simulink model "BolandLab3"  (R2024a)
settings: Solver=VariableStepAuto  StartTime=0.0  StopTime=100  RelTol=1e-3
libraries: simulink x1, dspsigops x1
settings Model: Creator=Test  LastModifiedBy=Test

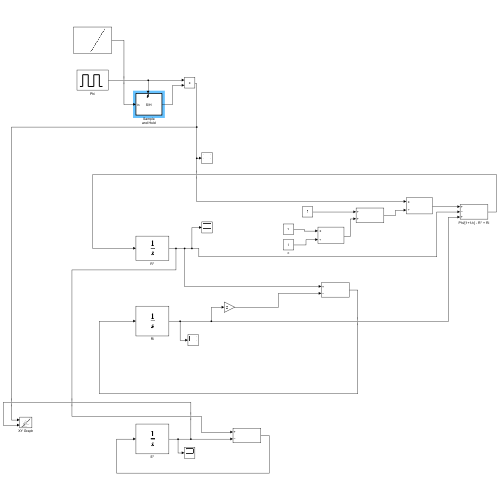
[thumbnail: Simulink's stored preview of the top-level diagram]
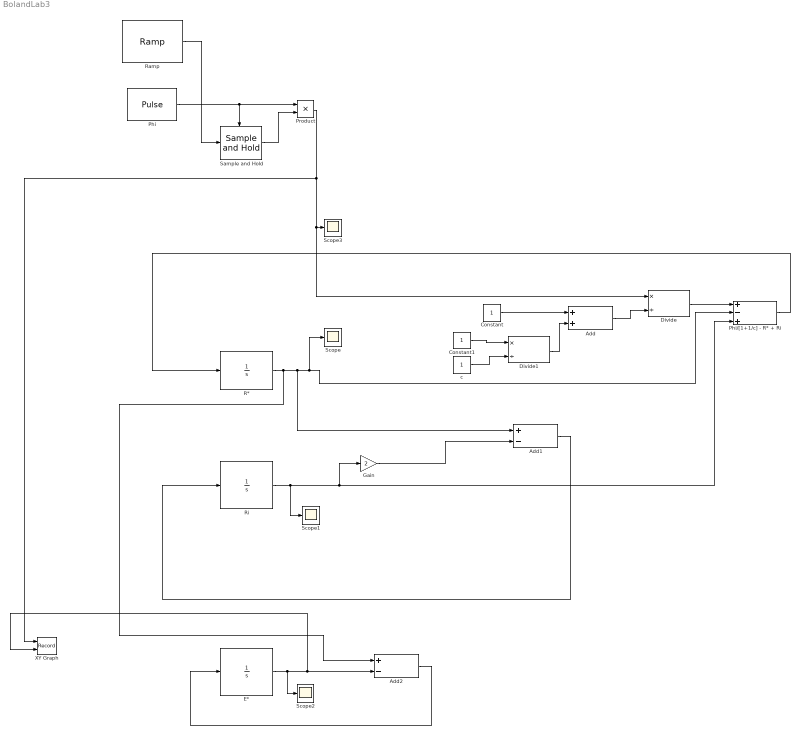
== system BolandLab3 ==
  Add : Sum
  Add1 : Sum  Inputs=+-
  Add2 : Sum  Inputs=+-
  Constant : Constant
  Constant1 : Constant
  Divide : Product  Inputs=*/
  Divide1 : Product  Inputs=*/
  E* : Integrator
  Gain : Gain  Gain=2
  Phi : DiscretePulseGenerator  PulseType=Time based  Period=10
  Phi/[1+1/c] - R* + Ri : Sum  Inputs=+-+
  Product : Product
  R* : Integrator
  Ramp : simulink/Sources/Ramp  slope=.1  start=0  InitialOutput=0
  Ri : Integrator
  Sample and Hold : dspsigops/Sample and Hold  trig=Rising edge  initCond=0  latchinput=off
  Scope{,1..3} (4 alike) : Scope
  XY Graph : Record  FileSettingsInternal="{\"entries\":[{\"content\":{\"excelSettings\":{\"content\":{},\"type\":\"Streamout.ExcelSettings\"}},\"type\":\"Streamout.FileSettingStorage\",\"uuid\":\"\"}],\"packageUris\":[\"http:\\/\\/schema.mathworks.com\\/mf0\\/streamout_blocks\\/R2020a\"],\"version\":\"1.0\"}"  Layout=[1 1]  SignalsInternal="{\"entries\":[{\"content\":{\"signals\":[{\"content\":{\"blockPath\":[],\"dimensions\":[1],\"domain\":\"\",\"lineColor\":\"#a2142f\",\"plots\":[ 1 ],\"port\":1,\"sid\":[\"\"],\"signalID\":1,\"signalName\":\"Product\"},\"type\":\"RecordBlkView.Signal\",\"uuid\":\"\"},{\"content\":{\"blockPath\":[],\"dimensions\":[1],\"domain\":\"\",\"lineColor\":\"#139fff\",\"plots\":[ 1 ],\"port\":2,\"sid\":[\"\"],\"signalID\":2,\"signalName\":\"E*\"},\"type\":\"RecordBlkView.Signal\",\"uuid\":\"\"}]},\"type\":\"RecordBlkView.InputSignals\",\"uuid\":\"\"}],\"packageUris\":[\"http:\\/\\/schema.mathworks.com\\/mf0\\/streamout_blocks\\/R2020a\"],\"version\":\"1.0\"}"  VisualizationBindings="{\"xyplotplugin\":{\"info\":[{\"series\":[{\"bindingParametersList\":[{\"parameter\":\"X-Axis\",\"signalID\":1,\"signalName\":\"Product\"},{\"parameter\":\"Y-Axis\",\"signalID\":2,\"signalName\":\"E*\"}],\"seriesID\":0}],\"subplotID\":1}]}}"  CompatibilityTag=XY
  c : Constant
  wires:
  Add/1 -> Divide/2
  Constant/1 -> Add/1
  Constant1/1 -> Divide1/1
  c/1 -> Divide1/2
  Divide1/1 -> Add/2
  Divide/1 -> Phi/[1+1/c] - R* + Ri/1
  Ri/1 -> Scope1/1, Gain/1, Phi/[1+1/c] - R* + Ri/3
  Phi/[1+1/c] - R* + Ri/1 -> R*/1
  Gain/1 -> Add1/2
  Add1/1 -> Ri/1
  E*/1 -> Scope2/1, XY Graph/2, Add2/2
  R*/1 -> Add2/1, Add1/1, Scope/1, Phi/[1+1/c] - R* + Ri/2
  Add2/1 -> E*/1
  Product/1 -> XY Graph/1, Divide/1, Scope3/1
  Phi/1 -> Sample and Hold/Trigger, Product/1
  Sample and Hold/1 -> Product/2
  Ramp/1 -> Sample and Hold/1
